simulink model "SABiR_simulator"  (Simulink 8.0)
settings: configuration reference "cset1" (kept outside this file)
values from neighbouring files (symbols this model uses):
  act_Lc_axis1 = act_Phi_axis1 \ acker(act_Phi_axis1', act_H_axis1', poles_Lpr1(1:length(act_Phi_axis1)) )'    [API_setupConstants.m]
  act_Lc_axis2 = act_Phi_axis2 \ acker(act_Phi_axis2', act_H_axis2', poles_Lpr2(1:length(act_Phi_axis2)) )'    [API_setupConstants.m]
  act_Lc_axis3 = act_Phi_axis3 \ acker(act_Phi_axis3', act_H_axis3', poles_Lpr3(1:length(act_Phi_axis3)) )'    [API_setupConstants.m]
  act_Lc_axis4 = act_Phi_axis4 \ acker(act_Phi_axis4', act_H_axis4', poles_Lpr4(1:length(act_Phi_axis4)) )'    [API_setupConstants.m]
  act_Lc_axis5 = act_Phi_axis5 \ acker(act_Phi_axis5', act_H_axis5', poles_Lpr5(1:length(act_Phi_axis5)) )'    [API_setupConstants.m]
  block1MinMax = [-20 0; -240 -180; 340 360]    [API_debugGraphs.m]    (also in API_setupConstants.m)
  block2MinMax = [-12 -7; -220 -200; 345 350]    [API_debugGraphs.m]    (also in API_setupConstants.m)
  est_Gamma_axis1 = [act_Gamma_axis1; 0]    [API_setupConstants.m]
  est_Gamma_axis2 = [act_Gamma_axis2; 0]    [API_setupConstants.m]
  est_Gamma_axis3 = [act_Gamma_axis3; 0]    [API_setupConstants.m]
  est_Gamma_axis4 = [act_Gamma_axis4; 0]    [API_setupConstants.m]
  est_Gamma_axis5 = [act_Gamma_axis5; 0]    [API_setupConstants.m]
  est_H_axis1 = [act_H_axis1, 0]    [API_setupConstants.m]
  est_H_axis2 = [act_H_axis2, 0]    [API_setupConstants.m]
  est_H_axis3 = [act_H_axis3, 0]    [API_setupConstants.m]
  est_H_axis4 = [act_H_axis4, 0]    [API_setupConstants.m]
  est_H_axis5 = [act_H_axis5, 0]    [API_setupConstants.m]
  est_Lc_axis1 = est_Phi_axis1 \ est_Lp_axis1    [API_setupConstants.m]
  est_Lc_axis2 = est_Phi_axis2 \ est_Lp_axis2    [API_setupConstants.m]
  est_Lc_axis3 = est_Phi_axis3 \ est_Lp_axis3    [API_setupConstants.m]
  est_Lc_axis4 = est_Phi_axis4 \ est_Lp_axis4    [API_setupConstants.m]
  est_Lc_axis5 = est_Phi_axis5 \ est_Lp_axis5    [API_setupConstants.m]
  est_Phi_axis1 = [act_Phi_axis1, act_Gamma_axis1; zeros(1,size(act_Phi_axis1,2)), 1]    [API_setupConstants.m]
  est_Phi_axis2 = [act_Phi_axis2, act_Gamma_axis2; zeros(1,size(act_Phi_axis2,2)), 1]    [API_setupConstants.m]
  est_Phi_axis3 = [act_Phi_axis3, act_Gamma_axis3; zeros(1,size(act_Phi_axis3,2)), 1]    [API_setupConstants.m]
  est_Phi_axis4 = [act_Phi_axis4, act_Gamma_axis4; zeros(1,size(act_Phi_axis4,2)), 1]    [API_setupConstants.m]
  est_Phi_axis5 = [act_Phi_axis5, act_Gamma_axis5; zeros(1,size(act_Phi_axis5,2)), 1]    [API_setupConstants.m]
  K_axis1 = acker(act_Phi_axis1, act_Gamma_axis1, poles_Kc1)    [API_setupConstants.m]
  K_axis2 = acker(act_Phi_axis2, act_Gamma_axis2, poles_Kc2)    [API_setupConstants.m]
  K_axis3 = acker(act_Phi_axis3, act_Gamma_axis3, poles_Kc3)    [API_setupConstants.m]
  K_axis4 = acker(act_Phi_axis4, act_Gamma_axis4, poles_Kc4)    [API_setupConstants.m]
  K_axis5 = acker(act_Phi_axis5, act_Gamma_axis5, poles_Kc5)    [API_setupConstants.m]
  Kd_dir = [0;0]    [API_setupConstants.m]
  Kd_pos = [0.0;0.0;0.0]    [API_setupConstants.m]
  Kdir = [12.5; 12.5]    [API_setupConstants.m]
  Kpos = [12.5; 12.5; 12.5]    [API_setupConstants.m]
  Nbar_axis1 = Nu_axis1 + K_axis1 * Nx_axis1    [API_setupConstants.m]
  Nbar_axis2 = Nu_axis2 + K_axis2 * Nx_axis2    [API_setupConstants.m]
  Nbar_axis3 = Nu_axis3 + K_axis3 * Nx_axis3    [API_setupConstants.m]
  Nbar_axis4 = Nu_axis4 + K_axis4 * Nx_axis4    [API_setupConstants.m]
  Nbar_axis5 = Nu_axis5 + K_axis5 * Nx_axis5    [API_setupConstants.m]
  SaturationLowerLimit = -[2;2;2;10;10;0.2]    [API_setupConstants.m]
  SaturationUpperLimit = [2;2;2;10;10;0.2]    [API_setupConstants.m]
  TorqueConstant = [TorqueConstantMotorRE25;     TorqueConstantMotorRE25;     TorqueConstantMotorRE30;     TorqueConstantMotorRE25;     TorqueConstantMotorRE25;     TorqueConstantMotorRE10]./GearRatio    [API_setupConstants.m]
  ts = 0.001    [API_relativeMove.m]    (also in API_setupConstants.m = 0.01; PosRef3D.m; PosRef3D_smooth.m; PosRefConfigSpace.m)
  ts2 = 0.0005    [API_setupConstants.m]
  tsEncoderFailure = TotalTime * encoderFailureTime    [API_simulateRobot.m]
undefined symbols (not defined in the file or in its folder): act_Gamma_axis1, act_Gamma_axis2, act_Gamma_axis3, act_Gamma_axis4, act_Gamma_axis5, act_H_axis1, act_H_axis2, act_H_axis3, act_H_axis4, act_H_axis5, act_Phi_axis1, act_Phi_axis2, act_Phi_axis3, act_Phi_axis4, act_Phi_axis5, den1, den2, den3, den4, den5, DiscIntNeverNeededParam, f_envfilt, J1_r, J2_r, J3_r, J4_r, J5_r, materialParameters1x, materialParameters2x, num1, num2, num3, num4, num5, numEncoderToFail
libraries: simulink x3
(part 3 of 3)

== matlab function forward kinematics/forward kinematics1 ==
  data: t1 input double; NeedleTip output double; NeedleRot output double; Front output double; t2 input double; t3 input double; t4 input double; t5 input double; Back output double; Jf output double; Jb output double
function [NeedleTip,NeedleRot,Front,Back,Jf,Jb]=SABiRFK(t1,t2,t3,t4,t5)
% function [NeedleTip,Rz,Front,Back]=SABiRFK(angles)

% SABiR Forward Kinematics
% Given angles in radians, returns end-effector and needle positions in mm.
% Usage: Needle_Tip_Position=SABiRFK([225,315,0,225,315].*pi./180)
%        [Needle_Tip_Position,R,Front,Back]=SABiRFK([225,315,0,225,315]*pi/180)
% Ozkan Bebek
% Modified syringe mechanism to match pb to pr on Nov/30/2009


% correct for the biases

t1bias= 225*pi/180;                      % Home position for axis 1
t2bias= 315*pi/180;                      % Home position for axis 2
t3bias= 0;                               % Home position for axis 3
t4bias= 225*pi/180;                      % Home position for axis 4
t5bias= 315*pi/180;                      % Home position for axis 5

t1 = t1 + t1bias;
t2 = t2 + t2bias;
t3 = t3 + t3bias;
t4 = t4 + t4bias;
t5 = t5 + t5bias;



%% Set up constants

%angular offset
alphax=0*pi/180;
alphay=0*pi/180;
R_BbBs=ypr2R(0,alphay,alphax,'rad');

yoffset=0;
xoffset=0;
zoffset=0;

ln= 68.6308+65.19+161.86+18.00+14.91;
ln1 = 123.142;
ln2=ln-ln1;
T_BackFront_mount = [ %July 22, 2010
    0.9996514523262   0.0239862420680  -0.0110287829636   -2.6398505898723
    -0.0238096717995   0.9995905085098   0.0158718249104  -45.1866546135221
    0.0114049722052  -0.0156037011200   0.9998132081146  197.5288079400060
    0                 0                 0                  1];

T_BackFront_mount_inv = [ T_BackFront_mount(1:3,1:3)', -T_BackFront_mount(1:3,1:3)'*T_BackFront_mount(1:3,4); 0 0 0 1];

%% Forward Kinematics Paramenters
% front stage
lf1=100;       %mm link length
lf2=100;       %mm link length
lfe=20.037 ;   %mm  end effector distance
zfgimbal=2.05; %mm offset

% back stage
lb1=100;       %mm link length
lb2=100;       %mm link length
lbe=65.532;    %mm  distance between end last joint of back stage and needle axis
zbgimbal=2.455; %mm offset

%% Front and back stage end points
xb=lb1*cos(t4)+lb2*cos(t5)+lbe*cos(t5-pi/4);
yb=(lb1*sin(t4)+lb2*sin(t5)+lbe*sin(t5-pi/4))*cos(-t3)-zbgimbal*sin(-t3);
zb=(lb1*sin(t4)+lb2*sin(t5)+lbe*sin(t5-pi/4))*sin(-t3)+zbgimbal*cos(-t3);
Back=[xb,yb,zb];

xb1=lb1*cos(t4)+lb2*cos(t5);
yb1=(lb1*sin(t4)+lb2*sin(t5))*cos(-t3)-zbgimbal*sin(-t3);
zb1=(lb1*sin(t4)+lb2*sin(t5))*sin(-t3)+zbgimbal*cos(-t3);
pb1=[xb1 yb1 zb1];

pf_front=[lf1*cos(t1)+lf2*cos(t2)+lfe*cos(t2-pi/4);
          lf1*sin(t1)+lf2*sin(t2)+lfe*sin(t2-pi/4);
          zfgimbal;
          1];
pf_back=T_BackFront_mount*pf_front;
Front=[pf_back(1),pf_back(2),pf_back(3)]; %=[xf,yf,zf]


%
% Tip point and needle direction calculations for the simplfied kinematics
% with alphax=alphay=0
%

% %% tip position of needle 
% k=Front-Back;
% t=ln/sqrt(sum(k.^2));
% % ignore offsets if don't exist
% if isempty(xoffset) && isempty(yoffset) && isempty(zoffset) 
% %     NeedleTip=t*k+Back;
%     nTip = t*k+Back;
% else
% %     NeedleTip=t*k+Back+[xoffset yoffset zoffset];    
%     nTip=t*k+Back+[xoffset yoffset zoffset];   
% end
% 
% NeedleTip = nTip';
% % NeedleTip = [1 1 1]';
% 
% %% Needle tip orientation
% % direction of needle
% pfb=pf_back(1:3)-Back';
% pfb=pfb./norm(pfb);
% Rz=pfb;

%
% Tip point and needle direction calculations for the complete kinematics
% with nonzero alphax and alphay
%


%% find R_BB1, R_B1Bb, R_BbBs (joint angles of passive joints)


beta=acos(([0;0;ln1]' * R_BbBs*[0;0;1])/ln1);
k=Front-Back;
PfPb=sqrt(sum(k.^2));
PsPf=ln1*cos(pi-beta)+sqrt(ln1*ln1*cos(pi-beta)*cos(pi-beta)-ln1*ln1+PfPb*PfPb);

Pb1Pf=sqrt(sum((Front-pb1).^2));

Bb_Pf=R_BbBs*[0;0;PsPf]+[0;0;ln1];
x=Bb_Pf(1);y=Bb_Pf(2);z=Bb_Pf(3);
lb1f=Pb1Pf;

% gammax : joint angle of 1st passive joint(pitch of syringe)(corrected 1/4/2011)

if y==0,
    gammax=acos((x*x+y*y+z*z+lbe*lbe-lb1f*lb1f)/2/z/lbe);
else
    gammax=atan2((-z*(z*lbe^2+y^2*z-z*lb1f^2+x^2*z+z^3+(-x^4*y^2-y^6-2*y^4*z^2-y^2*z^4-2*y^4*x^2+2*y^4*lb1f^2-y^2*lbe^4+2*y^4*lbe^2-y^2*lb1f^4+2*z^2*lbe^2*y^2+2*y^2*z^2*lb1f^2-2*y^2*z^2*x^2+2*y^2*x^2*lb1f^2-2*y^2*lbe^2*x^2+2*y^2*lbe^2*lb1f^2)^(1/2))/(z^2+y^2)+lbe^2+x^2+y^2+z^2-lb1f^2)/lbe/y,(z*lbe^2+y^2*z-z*lb1f^2+x^2*z+z^3+(-x^4*y^2-y^6-2*y^4*z^2-y^2*z^4-2*y^4*x^2+2*y^4*lb1f^2-y^2*lbe^4+2*y^4*lbe^2-y^2*lb1f^4+2*z^2*lbe^2*y^2+2*y^2*z^2*lb1f^2-2*y^2*z^2*x^2+2*y^2*x^2*lb1f^2-2*y^2*lbe^2*x^2+2*y^2*lbe^2*lb1f^2)^(1/2))/(z^2+y^2)/lbe);
end

R_BB1=[-sin(t5-pi/4), -cos(t5-pi/4), 0; cos(t5-pi/4)*cos(-t3), -sin(t5-pi/4)*cos(-t3), -sin(-t3); cos(t5-pi/4)*sin(-t3), -sin(t5-pi/4)*sin(-t3), cos(-t3)];
R_B2Bb=Rx(gammax-pi/2);

a=R_B2Bb*Bb_Pf;
b=R_BB1'*(Front'-Back');
c=inv([a(1) a(3);a(3) -a(1)])*[b(1);b(3)];
gammay=atan2(c(2),c(1)); % gammay : joint angle of 2nd passive joint(yaw of syringe) (corrected 1/4/2011)
R_B1B2=Ry(gammay);

R_BBb=R_BB1*R_B1B2*R_B2Bb;
R_BBs=R_BBb*R_BbBs;


%% tip position of needle 
ps=R_BBb*[0;0;ln1]+Back';
pn=R_BBs*[0;0;ln2]+ps;

if isempty(xoffset) && isempty(yoffset) && isempty(zoffset) 
    nt=[pn(1);pn(2);pn(3)];
else
    nt=[pn(1);pn(2);pn(3)]+[xoffset; yoffset; zoffset];    
end
NeedleTip=[nt(1);nt(2);nt(3)];

Rz=R_BBs(:,3);  % needle is pointing in the z-direction

NeedleRot=R_BBs;

%% Jacobian calculations
%
% Note that Jacobian calculations use the simplfied kinematics model
% with alphax=alphay=0
%


%calculate B_Bb_R, the rotation from the world frame to the back gimbal
%frame: B_Bb_R = B_Be_R * Be_B2_R * B2_Bb_R = B_Be_R * Rx(gammax-pi/2) * Ry(gammay)
%where gammax and gammay are the angles of the back gimbal

pf = Front';
pbe = Back';
pfpbe = norm(pf-pbe);

% R_BBe = [-sin(t5-pi/4)              -cos(t5-pi/4)           0;
%           cos(t5-pi/4)*cos(t3)  -sin(t5-pi/4)*cos(t3)    sin(t3);
%           -cos(t5-pi/4)*sin(t3)  sin(t5-pi/4)*sin(t3)    cos(t3)];
%       
% % R_BbBs = eye(3); %assume a perfect mounting of the needle
% 
% % pspf = ln1*cos(beta) + sqrt(ln2^2*cos(beta)^2-(ln1^2-pfpbe^2));
% 
% % k=1; %just any integer, i choose 1
% % Bb_xf=Bb_Pf(1);Bb_yf=Bb_Pf(2);Bb_zf=Bb_Pf(3);
% % A = Bb_yf;
% % B = Bb_zf;
% % Bb_pf = Bb_Bs_R * [0 0 pspf]' + [0 0 ln1];
% 
% 
% Rotx = [1 0 0;
%       0 cos(gammax-pi/2) -sin(gammax-pi/2);
%       0 sin(gammax-pi/2) cos(gammax-pi/2)];
% R_B2Bb = Rotx;
%   
% Roty = [1 0 0;
%       0 cos(gammay) -sin(gammay);
%       0 sin(gammay) cos(gammay)];
% R_BeB2 = Roty;
% 
% R_BBb = R_BBe * R_BeB2 * R_B2Bb;


%calculate back-stage jacobian
R = R_BBb;
P = pbe;
Phat = [0 -P(3) P(2);P(3) 0 -P(1);-P(2) P(1) 0];

RxTheta1 = [1 0 0;
            0 cos(t3)  sin(t3);
            0 -sin(t3) cos(t3)];
RzTheta2 = [cos(t4) -sin(t4) 0;
            sin(t4) cos(t4) 0
            0 0 1];
RzTheta3 = [cos(t5) -sin(t5) 0;
            sin(t5) cos(t5) 0
            0 0 1];

W = zeros(3,1);
u = RxTheta1*[0 0 1]';
v = RxTheta1 * (RzTheta2 * [lb1 0 0]');
W(1) = u(2)*v(3) - u(3)*v(2);
W(2) = u(3)*v(1) - u(1)*v(3);
W(3) = u(1)*v(2) - u(2)*v(1);
W = -W;
% W = -(cross(RxTheta1*[0 0 1]' , RxTheta1 * (RzTheta3 * [lb1 0 0]')));

Jb = [-R'*(Phat*[-1 0 0]'), -R'*W, R'*W - R'*Phat*RxTheta1*[0 0 1]'];
% Jb = [Jb;zeros(size(Jb))];

%calculate front-stage jacobian
g_FBf=T_BackFront_mount_inv*[R_BBs,pf; 0 0 0 1];
R = g_FBf(1:3,1:3);
P = g_FBf(1:3,4);
Phat = [0 -P(3) P(2);P(3) 0 -P(1);-P(2) P(1) 0];

RxTheta1 = eye(3);
RzTheta2 = [cos(t1) -sin(t1) 0;
            sin(t1) cos(t1) 0
            0 0 1];
RzTheta3 = [cos(t2) -sin(t2) 0;
            sin(t2) cos(t2) 0
            0 0 1];

W = zeros(3,1);
u = RxTheta1*[0 0 1]';
v = RxTheta1 * (RzTheta2 * [lf1 0 0]');
W(1) = u(2)*v(3) - u(3)*v(2);
W(2) = u(3)*v(1) - u(1)*v(3);
W(3) = u(1)*v(2) - u(2)*v(1);
W = -W;
% W = -(cross(RxTheta1*[0 0 1]' , RxTheta1 * (RzTheta3 * [lf1 0 0]')));

Jf = [-R'*(Phat*[-1 0 0]'), -R'*W, R'*W - R'*Phat*RxTheta1*[0 0 1]'];
% Jf = [Jf;zeros(size(Jf))];

== matlab function environment model/Needle force due to block 4/getForce ==
  data: pneedle input double; Rotneedle input double; blockMinMax input double; F_needle output double; T_needle output double; Matparametersx input double; depth output double; needleG output double; needleG_last input double; NormalWrench_Last input double; ts input double; NormalWrench output double
function [F_needle,T_needle,depth,needleG,NormalWrench] = getForce(pneedle,Rotneedle,blockMinMax,Matparametersx,needleG_last,NormalWrench_Last,ts)

Matparameters.mus=Matparametersx(1,1);
Matparameters.muk=Matparametersx(2,1);
Matparameters.K=Matparametersx(3:11,1);
Matparameters.alpha=Matparametersx(12,1);
Matparameters.limit=Matparametersx(13,1);

 

ln1 = 123.142;

blockMinMax = reshape(blockMinMax,3,2);


% %find the velocity of the needle
% pneedle_last = needleG_last * [0 0 ln1 1]';
% pneedle_last = pneedle_last(1:3);
% needleDiff = pneedle-pneedle_last;


%constant geometric parameters for straight needle (?)
Geoparameters = [0 0 0 0 0 0 0];

%needle is along the z-axis
rneedle=Rotneedle(1:3,3);

%now find the rotation matrix that rotates from base frame to needle frame
R = Rotneedle';

%transform R into quaternion form
Q = R2Q(R');

if( norm(R*R'-eye(3)) > 1e-12)
    error('R*Rt~=I.');
end

%create a needle struct for the Okamura force model

structNeedleGeometry = struct('straightL',ln1,'arc',0);
needlebase = pneedle - rneedle*ln1;
structNeedleData = struct('trans',needlebase,'rot',Q);
% block1MinMax = [-20 0; -240 -180; 340 360];
% block2MinMax = [-12 -7; -220 -200; 345 350]; 
structTissueData = struct('center',mean(blockMinMax'),'widthX',abs(blockMinMax(1,1)-blockMinMax(1,2)),'heightZ',abs(blockMinMax(3,1)-blockMinMax(3,2)),'depthY',abs(blockMinMax(2,1)-blockMinMax(2,2)));

N = 5; %number of points in needle 
[TissueState NeedlePtList]=Needle_Tissue_Intersection(structTissueData,structNeedleGeometry,structNeedleData,N);

structNeedleData_last = G2struct(needleG_last);
[TissueState_last NeedlePtList_last]=Needle_Tissue_Intersection(structTissueData,structNeedleGeometry,structNeedleData_last,N);

[wrenchModeled,wrenchFriction,wrenchNormal,wrenchCut] = Needle_Cumulative_Forces_Step(TissueState_last,NeedlePtList_last,TissueState,NeedlePtList,Matparameters,NormalWrench_Last);
% 
% wrenchModeled = zeros(6,1);
% wrenchFriction = zeros(6,1);
% wrenchNormal = zeros(6,1);
% wrenchCut = zeros(6,1);


L1 = NeedlePtList(1:3,2:N+1)-NeedlePtList(1:3,1:N);

L1a = L1'*L1;

L2 = diag(L1a);

L2a = (L2).^0.5;

depth = TissueState'*L2a; 

needleG= struct2G(structNeedleData);

if (depth == 0)
    F_needle=[0;0;0];
    T_needle=[0;0;0];
    NormalWrench=[0;0;0;0;0;0];
else
    depth = depth+L2a(1);
    NormalWrench=wrenchNormal;
    % %transform torques from world frame to needle frame
    % T_needle = R * T_needle - R * cross(needleTail, F_needle); 
    F_world = wrenchModeled(1:3);
    T_world = wrenchModeled(4:6);

    %transform forces from world frame to needle frame
    F_needle = R * F_world;

    %transform torques from world frame to needle frame
    T_needle = R * T_world - R * cross(pneedle, F_world); 
end

== matlab function convert environmental forces to joint torques/get joint torques ==
  data: F input double; T input double; Front input double; Back input double; torques output double; Jf input double; Jb input double
function torques = getTorques(F,T,Front,Back,Jf,Jb)

% set up A matrix

l1 = 328.5908;
l0 = norm(Front-Back);
l2 = l1-l0;

A = [1   0   0   1    0;
    0   1   0   0    1;
    0   0   1   0    0;
    0   l1  0   0    l2;
    -l1 0   0   -l2  0];

%% get Ft, the force/torque with respect to the needletip

% % for the straight needle with only axial force, b is simple
% Ft = [0 0 -f 0 0]';

%for the straight needle with non-axial forces, b is as follows

Ft = [F(1) F(2) F(3) T(1) T(2)]';

% get the forces at the gimbal joints
b=Ft;
x= A\b;

fbx = x(1);
fby = x(2);
fbz = x(3);
fcx = x(4);
fcy = x(5);

% get the front and back stage forces out of x

%add in the zero force to front-stage forces
Ff = [fcx fcy 0]';

%multiply by front-stage jacobian transpose
Tf = Jf'*Ff;

%multiply by back-stage jacobian transpose
Fb = [fbx fby fbz]';

Tb = Jb'*Fb;

torques = [Tf(2); Tf(3); Tb(1); Tb(2); Tb(3)];
